simulink model "PWMSignalAnalysis"  (R2014a)
settings: Solver=ode23t  StartTime=0.0  StopTime=1/input.fs*3  MaxStep=1e-3  MinStep=1e-12  RelTol=1e-3
undefined symbols (not defined in the file or in its folder): input
libraries: fl_lib x11, nesl_utility x10, powerlib_meascontrol x2
settings Model: Creator=sizuest  LastModifiedBy=simon
settings SolverCC: MaxConsecutiveMinStep=10
settings DataIOCC: SignalLoggingSaveFormat=ModelDataLogs
settings DebuggingCC: UnderspecifiedInitializationDetection=Classic  MaxConsecutiveZCsMsg=none  IgnoredZcDiagnostic=none  MultiTaskDSMMsg=warning  MultiTaskCondExecSysMsg=none  ParameterPrecisionLossMsg=none
settings RTWCC: IncludeERTFirstTime=on

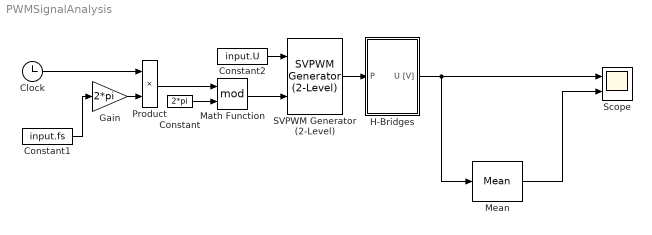
== system PWMSignalAnalysis ==
  Clock : Clock
  Constant : Constant  Value=2*pi
  Constant1 : Constant  Value=input.fs
  Constant2 : Constant  Value=input.U
  Gain : Gain  Gain=2*pi
  H-Bridges : Subsystem
  Math Function : Math  Operator=mod  SaturateOnIntegerOverflow=on
  Mean : powerlib_meascontrol/Measurements/Mean  Freq=pwm.f  Vinit=0  Ts=0
  Product : Product
  SVPWM Generator (2-Level) : powerlib_meascontrol/Pulse & Signal Generators/SVPWM Generator (2-Level)  InputType=Magnitude-Angle (rad)  SwitchingPattern=Pattern #1  Fc=pwm.f  ParUref=[10/400 0 3.7]  Ts=0
  Scope : Scope  NumInputPorts=2
      settings: YMin=-2.75e-14~-1.5e-14  YMax=2.75e-14~1.5e-14  SaveName=ScpPWM  SampleInput=on  SampleTime=1/pwm.f/20
  wires:
  H-Bridges/1(U [V]) -> Mean/1, Scope/1
  Mean/1 -> Scope/2
  SVPWM Generator (2-Level)/1 -> H-Bridges/1(P)
  Constant1/1 -> Gain/1
  Clock/1 -> Product/1
  Gain/1 -> Product/2
  Product/1 -> Math Function/1
  Constant/1 -> Math Function/2
  Constant2/1 -> SVPWM Generator (2-Level)/1
  Math Function/1 -> SVPWM Generator (2-Level)/2

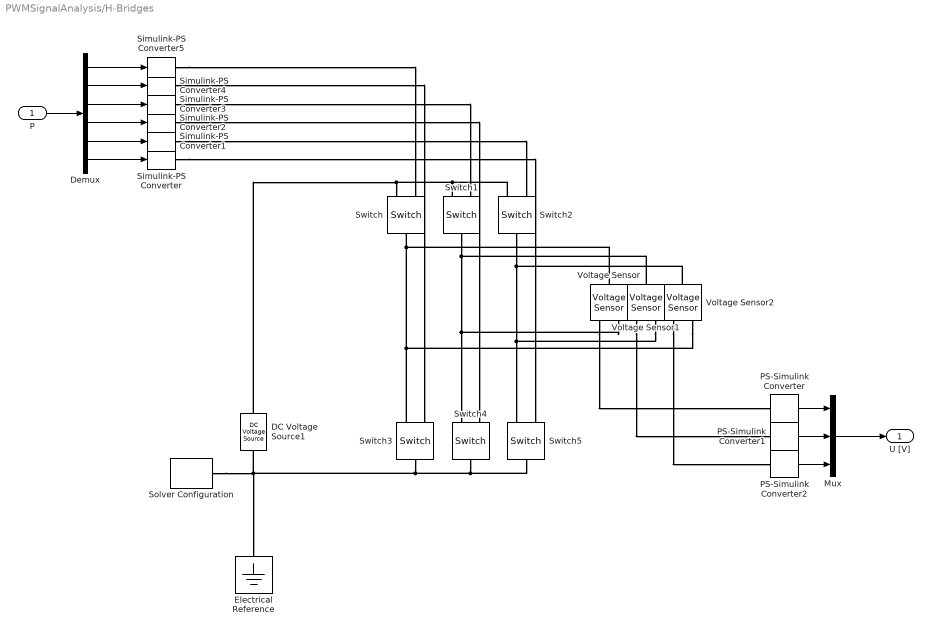
== system PWMSignalAnalysis/H-Bridges ==
  P : Inport
  DC Voltage Source1 : fl_lib/Electrical/Electrical Sources/DC Voltage Source  v0=pwm.Umax V
  Demux : Demux  Outputs=6
  Electrical Reference : fl_lib/Electrical/Electrical Elements/Electrical Reference
  Mux : Mux  Inputs=3
  PS-Simulink Converter : nesl_utility/PS-Simulink Converter  PhysicalDomain=network_engine_domain  SubClassName=ps_output  LeftPortType=input  RightPortType=output  PseudoPeriodic=off  Frequencies=[]  Unit=1  AffineConversion=off
  PS-Simulink Converter1 : nesl_utility/PS-Simulink Converter  PhysicalDomain=network_engine_domain  SubClassName=ps_output  LeftPortType=input  RightPortType=output  PseudoPeriodic=off  Frequencies=[]  Unit=1  AffineConversion=off
  PS-Simulink Converter2 : nesl_utility/PS-Simulink Converter  PhysicalDomain=network_engine_domain  SubClassName=ps_output  LeftPortType=input  RightPortType=output  PseudoPeriodic=off  Frequencies=[]  Unit=1  AffineConversion=off
  Simulink-PS Converter{,1..5} (6 alike) : nesl_utility/Simulink-PS Converter  PhysicalDomain=network_engine_domain  SubClassName=ps_input  LeftPortType=input  RightPortType=output  PseudoPeriodic=off  Frequencies=[]  NoiseDistribution=none  NoiseParameters=[]  Unit=1  AffineConversion=off  InputFiltering=off  SimscapeFilterOrder=1  InputFilterTimeConstant=0.001  UdotUserProvided=1
  Solver Configuration : nesl_utility/Solver Configuration  PhysicalDomain=network_engine_domain  SubClassName=solver  LeftPortType=input  RightPortType=generic  Accelerate=off  Tones=[]  Harmonics=[]  SimulateNoise=off  Profile=off  UseLocalSampling=off  EnableSwitchedLinearOptims=on  FrequencyDomain=off  UseCCode=off  RelTol=0.001  AbsTol=1e-06  MinStep=1e-09  ToWorkspace=off  DoDC=off  ResidualTolerance=1e-09  UseLocalSolver=off  LocalSolverChoice=NE_BACKWARD_EULER_ADVANCER  LocalSolverSampleTime=0.001  DoFixedCost=off  MaxNonlinIter=3  MaxModeIter=2  LinearAlgebra=Sparse  DelaysMemoryBudget=1024  AutomaticFiltering=on  FilteringTimeConstant=0.001
  Switch{,1..5} (6 alike) : fl_lib/Electrical/Electrical Elements/Switch  R_closed=0.01 Ohm  G_open=1e-8 1/Ohm  Threshold=0  i_specify=off  i_priority=High  i=0 A  v_specify=off  v_priority=High  v=0 V
  Voltage Sensor : fl_lib/Electrical/Electrical Sensors/Voltage Sensor
  Voltage Sensor1 : fl_lib/Electrical/Electrical Sensors/Voltage Sensor
  Voltage Sensor2 : fl_lib/Electrical/Electrical Sensors/Voltage Sensor
  U [V] : Outport
  wires:
  PS-Simulink Converter2/1 -> Mux/3
  PS-Simulink Converter1/1 -> Mux/2
  PS-Simulink Converter/1 -> Mux/1
  Mux/1 -> U [V]/1
  P/1 -> Demux/1
  Demux/1 -> Simulink-PS Converter5/1
  Demux/2 -> Simulink-PS Converter4/1
  Demux/3 -> Simulink-PS Converter3/1
  Demux/4 -> Simulink-PS Converter2/1
  Demux/5 -> Simulink-PS Converter1/1
  Demux/6 -> Simulink-PS Converter/1
  connections:
  Switch/RConn2 -- DC Voltage Source1/LConn1 -- Switch1/RConn2 -- Switch2/RConn2
  Switch/LConn1 -- Voltage Sensor2/RConn2 -- Switch3/RConn2 -- Voltage Sensor/LConn1
  Switch1/LConn1 -- Voltage Sensor1/LConn1 -- Voltage Sensor/RConn2 -- Switch4/RConn2
  Switch2/LConn1 -- Voltage Sensor2/LConn1 -- Voltage Sensor1/RConn2 -- Switch5/RConn2
  Solver Configuration/RConn1 -- Electrical Reference/LConn1 -- DC Voltage Source1/RConn1 -- Switch3/LConn1 -- Switch5/LConn1 -- Switch4/LConn1
  Simulink-PS Converter5/RConn1 -- Switch/RConn1
  Simulink-PS Converter4/RConn1 -- Switch3/RConn1
  Simulink-PS Converter3/RConn1 -- Switch1/RConn1
  Simulink-PS Converter2/RConn1 -- Switch4/RConn1
  Simulink-PS Converter1/RConn1 -- Switch2/RConn1
  Simulink-PS Converter/RConn1 -- Switch5/RConn1
  Voltage Sensor/RConn1 -- PS-Simulink Converter/LConn1
  Voltage Sensor1/RConn1 -- PS-Simulink Converter1/LConn1
  Voltage Sensor2/RConn1 -- PS-Simulink Converter2/LConn1
